simulink model "naibaoDSTBC_22"  (R2018a)
settings: Solver=VariableStepAuto  StartTime=0.0  StopTime=10  RelTol=1e-3
model workspace (MAT data in the model file):
  FrameLength = 100
  SampleTime = 0.001
  maxNumBits = 100000000
  maxNumErrs = 1000
undefined symbols (not defined in the file): doppler
libraries: commchan3 x5, commrandsrc3 x1, commsink2 x1, commmimo x1
settings Model: Creator=myste  LastModifiedBy=myste

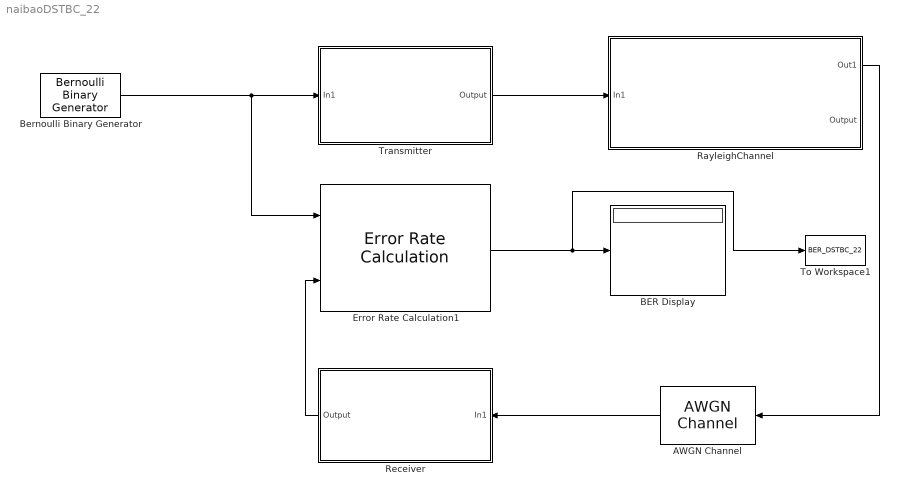
== system naibaoDSTBC_22 ==
  AWGN Channel : commchan3/AWGN Channel  InputProcessing=Columns as channels (frame based)  seed=67  noiseMode="Signal to noise ratio  (Eb/No)"  EbNodB=EbNo  EsNodB=10  SNRdB=10  bitsPerSym=1  Ps=1  Tsym=SampleTime  variance=1
  BER Display : Display
  Bernoulli Binary Generator : commrandsrc3/Bernoulli Binary Generator  ProbabilityOfZero=0.5  SeedSource=Auto  Seed=1983  SampleTime=SampleTime  SamplesPerFrame=FrameLength  OutputDataType=boolean  SimulateUsing=Interpreted execution
  Error Rate Calculation1 : commsink2/Error Rate Calculation  N=0  st_delay=0  cp_mode=Entire frame  subframe=[]  PMode=Port  WsName=ErrorVec  RsMode2=off  stop=on  numErr=maxNumErrs  maxBits=maxNumBits
  RayleighChannel : Subsystem
  Receiver : Subsystem
  To Workspace1 : ToWorkspace  VariableName=BER_DSTBC_22  SampleTime=-1
      settings: MaxDataPoints=1  Save2DSignal=2-D array (concatenate along first dimension)
  Transmitter : Subsystem
  wires:
  Error Rate Calculation1/1 -> To Workspace1/1, BER Display/1
  Bernoulli Binary Generator/1 -> Error Rate Calculation1/1, Transmitter/1(In1)
  Transmitter/1(Output) -> RayleighChannel/1(In1)
  RayleighChannel/1(Out1) -> AWGN Channel/1
  AWGN Channel/1 -> Receiver/1(In1)
  Receiver/1(Output) -> Error Rate Calculation1/2

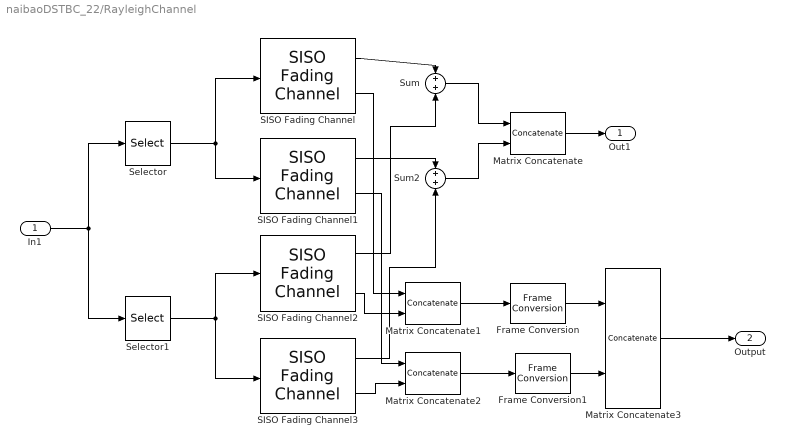
== system naibaoDSTBC_22/RayleighChannel ==
  In1 : Inport
  Frame Conversion : FrameConversion  OutFrame=Sample-based
  Frame Conversion1 : FrameConversion  OutFrame=Sample-based
  Matrix Concatenate : Concatenate  Mode=Multidimensional array  ConcatenateDimension=2
  Matrix Concatenate1 : Concatenate  Mode=Multidimensional array  ConcatenateDimension=2
  Matrix Concatenate2 : Concatenate  Mode=Multidimensional array  ConcatenateDimension=2
  Matrix Concatenate3 : Concatenate  Mode=Multidimensional array  ConcatenateDimension=3
  SISO Fading Channel : commchan3/SISO Fading Channel  InheritSampleRate=on  SampleRate=1  PathDelays=0  AveragePathGains=0  NormalizePathGains=on  FadingDistribution=Rayleigh  KFactor=3  DirectPathDopplerShift=0  DirectPathInitialPhase=0  MaximumDopplerShift=3  DopplerSpectrum=doppler('Jakes')  ChannelInterpolationMethod=Polyphase  RandomStream=mt19937ar with seed  RandomNumGenerator=mt19937ar  Seed=123  PathGainsOutputPort=on  ChannelFilterDelayOutputPort=off  SimulateUsing=Interpreted execution  Visualization=Off  PathsForDopplerDisplay=1  SamplesToDisplay=25%
      settings: SourceProductName=Communications System Toolbox
  SISO Fading Channel1 : commchan3/SISO Fading Channel  InheritSampleRate=on  SampleRate=1  PathDelays=0  AveragePathGains=0  NormalizePathGains=on  FadingDistribution=Rayleigh  KFactor=3  DirectPathDopplerShift=0  DirectPathInitialPhase=0  MaximumDopplerShift=3  DopplerSpectrum=doppler('Jakes')  ChannelInterpolationMethod=Polyphase  RandomStream=mt19937ar with seed  RandomNumGenerator=mt19937ar  Seed=73  PathGainsOutputPort=on  ChannelFilterDelayOutputPort=off  SimulateUsing=Interpreted execution  Visualization=Off  PathsForDopplerDisplay=1  SamplesToDisplay=25%
      settings: SourceProductName=Communications System Toolbox
  SISO Fading Channel2 : commchan3/SISO Fading Channel  InheritSampleRate=on  SampleRate=1  PathDelays=0  AveragePathGains=0  NormalizePathGains=on  FadingDistribution=Rayleigh  KFactor=3  DirectPathDopplerShift=0  DirectPathInitialPhase=0  MaximumDopplerShift=3  DopplerSpectrum=doppler('Jakes')  ChannelInterpolationMethod=Polyphase  RandomStream=mt19937ar with seed  RandomNumGenerator=mt19937ar  Seed=88  PathGainsOutputPort=on  ChannelFilterDelayOutputPort=off  SimulateUsing=Interpreted execution  Visualization=Off  PathsForDopplerDisplay=1  SamplesToDisplay=25%
      settings: SourceProductName=Communications System Toolbox
  SISO Fading Channel3 : commchan3/SISO Fading Channel  InheritSampleRate=on  SampleRate=1  PathDelays=0  AveragePathGains=0  NormalizePathGains=on  FadingDistribution=Rayleigh  KFactor=3  DirectPathDopplerShift=0  DirectPathInitialPhase=0  MaximumDopplerShift=3  DopplerSpectrum=doppler('Jakes')  ChannelInterpolationMethod=Polyphase  RandomStream=mt19937ar with seed  RandomNumGenerator=mt19937ar  Seed=95  PathGainsOutputPort=on  ChannelFilterDelayOutputPort=off  SimulateUsing=Interpreted execution  Visualization=Off  PathsForDopplerDisplay=1  SamplesToDisplay=25%
      settings: SourceProductName=Communications System Toolbox
  Selector : Selector  NumberOfDimensions=2  InputPortWidth=3  IndexOptions=Select all,Index vector (dialog)  Indices=[1 3],1  OutputSizes=1,1
  Selector1 : Selector  NumberOfDimensions=2  InputPortWidth=3  IndexOptions=Select all,Index vector (dialog)  Indices=[1 3],2  OutputSizes=1,1
  Sum : Sum
  Sum2 : Sum
  Out1 : Outport
  Output : Outport  Port=2
  wires:
  In1/1 -> Selector1/1, Selector/1
  Selector/1 -> SISO Fading Channel/1, SISO Fading Channel1/1
  Selector1/1 -> SISO Fading Channel3/1, SISO Fading Channel2/1
  SISO Fading Channel/1 -> Sum/1
  SISO Fading Channel2/1 -> Sum/2
  SISO Fading Channel1/1 -> Sum2/1
  Sum/1 -> Matrix Concatenate/1
  Sum2/1 -> Matrix Concatenate/2
  SISO Fading Channel/2 -> Matrix Concatenate1/1
  SISO Fading Channel3/1 -> Sum2/2
  SISO Fading Channel2/2 -> Matrix Concatenate1/2
  SISO Fading Channel1/2 -> Matrix Concatenate2/1
  SISO Fading Channel3/2 -> Matrix Concatenate2/2
  Matrix Concatenate/1 -> Out1/1
  Matrix Concatenate1/1 -> Frame Conversion/1
  Matrix Concatenate2/1 -> Frame Conversion1/1
  Frame Conversion1/1 -> Matrix Concatenate3/2
  Frame Conversion/1 -> Matrix Concatenate3/1
  Matrix Concatenate3/1 -> Output/1

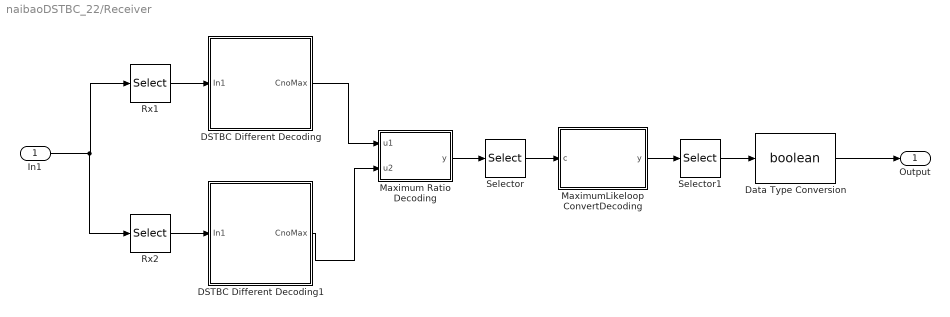
== system naibaoDSTBC_22/Receiver ==
  In1 : Inport
  DSTBC Different Decoding : Subsystem
  DSTBC Different Decoding1 : Subsystem
  Data Type Conversion : DataTypeConversion  OutDataTypeStr=boolean
  Maximum Ratio Decoding : MATLAB Function  TreatAsAtomicUnit=on
  MaximumLikeloop ConvertDecoding : MATLAB Function  TreatAsAtomicUnit=on
  Rx1 : Selector  NumberOfDimensions=2  InputPortWidth=3  IndexOptions=Select all,Index vector (dialog)  Indices=[1 3],1  OutputSizes=1,1
  Rx2 : Selector  NumberOfDimensions=2  InputPortWidth=3  IndexOptions=Select all,Index vector (dialog)  Indices=[1 3],2  OutputSizes=1,1
  Selector : Selector  NumberOfDimensions=2  InputPortWidth=3  IndexOptions=Select all,Index vector (dialog)  Indices=[1 3],1  OutputSizes=1,1
  Selector1 : Selector  NumberOfDimensions=2  InputPortWidth=3  IndexOptions=Select all,Index vector (dialog)  Indices=[1 3],1  OutputSizes=1,1
  Output : Outport
  wires:
  In1/1 -> Rx2/1, Rx1/1
  Rx1/1 -> DSTBC Different Decoding/1(In1)
  Rx2/1 -> DSTBC Different Decoding1/1(In1)
  Maximum Ratio Decoding/1(y) -> Selector/1
  DSTBC Different Decoding/1(CnoMax) -> Maximum Ratio Decoding/1(u1)
  DSTBC Different Decoding1/1(CnoMax) -> Maximum Ratio Decoding/2(u2)
  Data Type Conversion/1 -> Output/1
  Selector/1 -> MaximumLikeloop ConvertDecoding/1(c)
  MaximumLikeloop ConvertDecoding/1(y) -> Selector1/1
  Selector1/1 -> Data Type Conversion/1

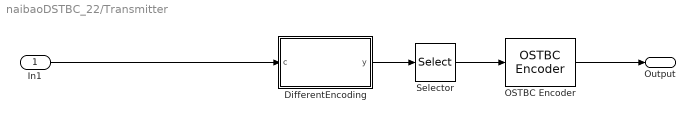
== system naibaoDSTBC_22/Transmitter ==
  In1 : Inport
  DifferentEncoding : MATLAB Function  TreatAsAtomicUnit=on
  OSTBC Encoder : commmimo/OSTBC Encoder  numTx=2  rate=3/4  overflowMode=Wrap  OvFlMode=off  OvFlModeLastStrValue=off
      settings: SourceProductName=Communications System Toolbox  SourceProductBaseCode=CM
  Selector : Selector  NumberOfDimensions=2  InputPortWidth=3  IndexOptions=Select all,Index vector (dialog)  Indices=[1 3],1  OutputSizes=1,1
  Output : Outport
  wires:
  OSTBC Encoder/1 -> Output/1
  Selector/1 -> OSTBC Encoder/1
  DifferentEncoding/1(y) -> Selector/1
  In1/1 -> DifferentEncoding/1(c)

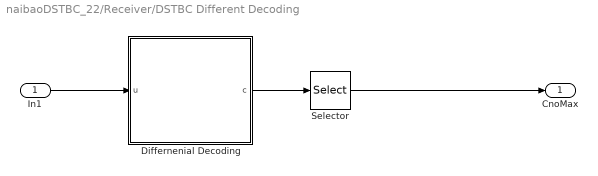
== system naibaoDSTBC_22/Receiver/DSTBC Different Decoding ==
  In1 : Inport
  Differnenial Decoding : MATLAB Function  TreatAsAtomicUnit=on
  Selector : Selector  NumberOfDimensions=2  InputPortWidth=3  IndexOptions=Select all,Index vector (dialog)  Indices=[1 3],1  OutputSizes=1,1
  CnoMax : Outport
  wires:
  In1/1 -> Differnenial Decoding/1(u)
  Differnenial Decoding/1(c) -> Selector/1
  Selector/1 -> CnoMax/1

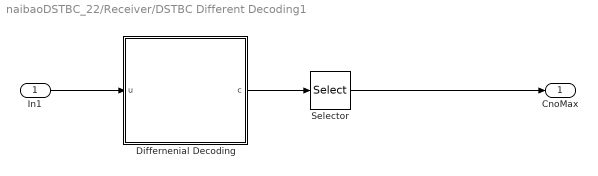
== system naibaoDSTBC_22/Receiver/DSTBC Different Decoding1 ==
  In1 : Inport
  Differnenial Decoding : MATLAB Function  TreatAsAtomicUnit=on
  Selector : Selector  NumberOfDimensions=2  InputPortWidth=3  IndexOptions=Select all,Index vector (dialog)  Indices=[1 3],1  OutputSizes=1,1
  CnoMax : Outport
  wires:
  Differnenial Decoding/1(c) -> Selector/1
  Selector/1 -> CnoMax/1
  In1/1 -> Differnenial Decoding/1(u)

== matlab function naibaoDSTBC_22/Receiver/DSTBC Different Decoding1/Differnenial Decoding ==
  data: u input; c output
function c = DifferenialDecode(u)
%% 基本参数
%获取帧长
s = size(u);
%分组块数
block = ( s(1)-2 ) /2;
%当前的接受信号Current_S1,Current_S2
current_S1 = u(1);
current_S2 = u(2);
%C1,C2
c1 = complex(zeros(block,2));
c2 = complex(zeros(block,2));
%输出序列C
c = complex(zeros(s(1)-2,2));
%% 循环实现
for i=1:block
    %编写信号X1,X2,X3
    X1=[current_S1,current_S2'];
    X3=[u(2*i+1,1),u(2*i+2,1)'];
    X2=[current_S2,-current_S1'];
    %得到差分码
    c1(i,1) = X3*X1';
    c2(i,1) = X3*X2';
    c(2*i-1,1) = c1(i,1);
    c(2*i,1)   = c2(i,1);
    current_S1 = u(2*i+1);
    current_S2 = u(2*i+2);
end
%% 输出

== matlab function naibaoDSTBC_22/Transmitter/DifferentEncoding ==
  data: c input; y output
function y= DifferentEncoding(c)
%% 设置参数
%得到帧长
s = size(c);
%计算BPSK的长度
BPSK_Len = s(1);
%初始化系数序列
u = complex(zeros(BPSK_Len,1));
%初始编码
current_S1 = 1/sqrt(2)+0i;
current_S2 = 1/sqrt(2)+0i;
%初始化发送信号序列
y=complex(zeros(BPSK_Len+2,2));
y(1,1)=current_S1;
y(2,1)=current_S2;
%% 差分编码
for i=1:BPSK_Len/2
    %计算得到系数
    ctemp=[c(2*i-1),c(2*i)];
    if ctemp == [0,0]
            u(2*i-1)=1;
            u(2*i)=0;
    else
        if ctemp==[1,0]
            u(2*i-1)=0;
            u(2*i)=1;
        else
            if ctemp==[0,1]
                u(2*i-1)=0;
                u(2*i)=-1;  
            else
                if ctemp==[1,1]
                    u(2*i-1)=-1;
                    u(2*i)=0;    
                end
            end
        end
    end
%得到向量基底 
    St1=[current_S1,current_S2];
    St2=[-current_S2',current_S1'];
%编码
	y(2*i+1,1) = u(2*i-1) * St1(1)+ u(2*i) * St2(1);
    y(2*i+2,1) = u(2*i-1) * St1(2)+ u(2*i) * St2(2);
%更改当前编码序列
    current_S1=y(2*i+1,1);
    current_S2=y(2*i+2,1);
end

== matlab function naibaoDSTBC_22/Receiver/DSTBC Different Decoding/Differnenial Decoding ==
  data: u input; c output
function c = DifferenialDecode(u)
%% 基本参数
%获取帧长
s = size(u);
%分组块数
block = ( s(1)-2 ) /2;
%当前的接受信号Current_S1,Current_S2
current_S1 = u(1);
current_S2 = u(2);
%C1,C2
c1 = complex(zeros(block,2));
c2 = complex(zeros(block,2));
%输出序列C
c = complex(zeros(s(1)-2,2));
%% 循环实现
for i=1:block
    %编写信号X1,X2,X3
    X1=[current_S1,current_S2'];
    X3=[u(2*i+1,1),u(2*i+2,1)'];
    X2=[current_S2,-current_S1'];
    %得到差分码
    c1(i,1) = X3*X1';
    c2(i,1) = X3*X2';
    c(2*i-1,1) = c1(i,1);
    c(2*i,1)   = c2(i,1);
    current_S1 = u(2*i+1);
    current_S2 = u(2*i+2);
end
%% 输出

== matlab function naibaoDSTBC_22/Receiver/Maximum Ratio Decoding ==
  data: u1 input; y output; u2 input
function y = mrd(u1,u2)
%两条信道完全对称,直接等增益合并
s=size(u1);
y=complex( zeros(s(1),2));
for i=1:s(1)
    y(i,1)=(u1(i)+u2(i))/2;
end

== matlab function naibaoDSTBC_22/Receiver/MaximumLikeloop ConvertDecoding ==
  data: c input; y output
function y  = MLC(c)
% 最大似然译码+逆映射
% 获取帧长
s=size(c);
FrameLen=s(1);
%初始化y
y=zeros(FrameLen,2);
%% 最大似然译码+逆映射
% 许用码字
allowcode=[ 1,0 ; 0,1 ; -1,0 ; 0,-1 ];
len=complex(zeros(4,1));
for i=1:FrameLen/2
    temp=[0+0i,1];
    if abs(c(2*i-1))>abs(c(2*i))
        c(2*i)=0;
    else 
        c(2*i-1)=0;
    end
    for j=1:4
        len(j)=c(2*i-1)'*allowcode(j,1)+...
                    c(2*i)'*allowcode(j,2); 
        if j==1 
            temp(1)=len(j);
        else
            if len(j)>temp(1)
                temp=[len(j),j];
            end
        end
    end
    c(2*i-1)=allowcode(temp(2),1);
    c(2*i)=allowcode(temp(2),2);
    
    if [c(2*i-1),c(2*i)]==[1,0]
        y(2*i-1,1)=0;
        y(2*i,1)=0;
    end
    if [c(2*i-1),c(2*i)]== [0,1]
        y(2*i-1,1)=1;
        y(2*i,1)=0;
    end
    if [c(2*i-1),c(2*i)]==[0,-1]
        y(2*i-1,1)=0;
        y(2*i,1)=1;
    end
    if [c(2*i-1),c(2*i)]==[-1,0]
        y(2*i-1,1)=1;
        y(2*i,1)=1;
    end
end
